simulink model "instrumentation_amplifier"  (R2020b)
settings: Solver=ode23t  StartTime=0.0  StopTime=4  RelTol=1e-3  EnableMultiTasking=on
libraries: fl_lib x10, ee_lib x7, nesl_utility x2
settings Model: Creator=lenovo  LastModifiedBy=bolic
settings DataIOCC: LimitDataPoints=on  SaveFormat=Array  SignalLoggingSaveFormat=ModelDataLogs  ReturnWorkspaceOutputs=off
settings OptimizationCC: ExpressionDepthLimit=2147483647  LifeSpan=inf
settings DebuggingCC: UnderspecifiedInitializationDetection=Classic  MergeDetectMultiDrivingBlocksExec=none  SolverPrmCheckMsg=warning  FcnCallInpInsideContextMsg=warning  StateNameClashWarn=warning  SFUnexpectedBacktrackingDiag=warning  SFNoUnconditionalDefaultTransitionDiag=warning  SFExecutionAtInitializationDiag=none  ArithmeticOperatorsInVariantConditions=warning
settings HardwareCC: ProdBitPerPointer=32  ProdBitPerSizeT=32  ProdBitPerPtrDiffT=32  ProdLargestAtomicFloat=None  ProdIntDivRoundTo=Undefined  ProdEndianess=Unspecified  ProdWordSize=32  ProdHWDeviceType=32-bit Generic
settings ModelReferenceCC: PropagateSignalLabelsOutOfModel=off
settings SFSimCC: SimUseLocalCustomCode=off  CustomCodeUndefinedFunction=UseInterfaceOnly
settings RTWCC: RTWUseLocalCustomCode=off
settings CodeAppCC: StateflowObjectComments=on
settings GRTTargetCC: TargetLangStandard=C89/C90 (ANSI)  CombineOutputUpdateFcns=off  GRTInterface=on
settings ConfigComp: CovMetricSettings=dw  CovSaveCumulativeToWorkspaceVar=on  CovSaveSingleToWorkspaceVar=on  CovExternalEMLEnable=off
settings SimscapeCC: SimscapeNormalizeSystem=off

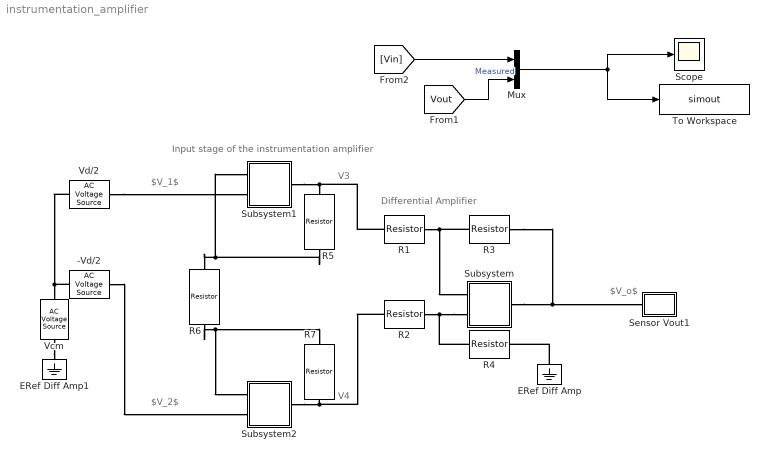
== system instrumentation_amplifier ==
  note: V4
  note: V3
  note: $V_o$
  note: Differential Amplifier
  note: Input stage of the instrumentation amplifier
  note: $V_1$
  note: $V_2$
  -Vd/2 : fl_lib/Electrical/Electrical Sources/AC Voltage Source  amp=0.02 V  shift=0 deg  frequency=1.2 Hz  omega=0 rad/s
  ERef Diff Amp : fl_lib/Electrical/Electrical Elements/Electrical Reference
      settings: SourceProductName=Foundation Library
  ERef Diff Amp1 : fl_lib/Electrical/Electrical Elements/Electrical Reference
      settings: SourceProductName=Foundation Library
  Mux : Mux  Inputs=2
  R1 : ee_lib/Passive/Resistor  R=1 kOhm  R_tol=1  enable_R_tol=0  tol_distribution=1  nSigma=4  enable_operating_limits=0  operating_limit_action=2  max_working_voltage=100 V  power_rating=1 W  enable_faults=0  fault_action=1  R_faulted=Inf Ohm  enable_temporal_fault=0  t_fault=1 s  enable_behavioral_fault=0  max_permissible_current=1 A  t_fail_on_current=1 s  noise_mode=0  sample_time=0.001 s  repeatability=1  auto_seed=2482559993  user_seed=0  Tdevice=25 degC  alpha=3.93e-3 1/K  Tmeas=25 degC  thermal_mass=100 J/K  power_derating_T1=70 degC  power_derating_T2=155 degC  operating_temperature_range_vec=[-50, 150] degC  temperature_specify=off  temperature_priority=High  temperature=298.15 K  temperature_nominal_specify=off  temperature_nominal_unit=K  temperature_nominal_value=1
  R2 : ee_lib/Passive/Resistor  R=1 kOhm  R_tol=1  enable_R_tol=0  tol_distribution=1  nSigma=4  enable_operating_limits=0  operating_limit_action=2  max_working_voltage=100 V  power_rating=1 W  enable_faults=0  fault_action=1  R_faulted=Inf Ohm  enable_temporal_fault=0  t_fault=1 s  enable_behavioral_fault=0  max_permissible_current=1 A  t_fail_on_current=1 s  noise_mode=0  sample_time=0.001 s  repeatability=1  auto_seed=854004048  user_seed=0  Tdevice=25 degC  alpha=3.93e-3 1/K  Tmeas=25 degC  thermal_mass=100 J/K  power_derating_T1=70 degC  power_derating_T2=155 degC  operating_temperature_range_vec=[-50, 150] degC  temperature_specify=off  temperature_priority=High  temperature=298.15 K  temperature_nominal_specify=off  temperature_nominal_unit=K  temperature_nominal_value=1
  R3 : ee_lib/Passive/Resistor  R=1 kOhm  R_tol=0.5  enable_R_tol=0  tol_distribution=1  nSigma=4  enable_operating_limits=0  operating_limit_action=2  max_working_voltage=100 V  power_rating=1 W  enable_faults=0  fault_action=1  R_faulted=Inf Ohm  enable_temporal_fault=0  t_fault=1 s  enable_behavioral_fault=0  max_permissible_current=1 A  t_fail_on_current=1 s  noise_mode=0  sample_time=0.001 s  repeatability=1  auto_seed=997392218  user_seed=0  Tdevice=25 degC  alpha=3.93e-3 1/K  Tmeas=25 degC  thermal_mass=100 J/K  power_derating_T1=70 degC  power_derating_T2=155 degC  operating_temperature_range_vec=[-50, 150] degC  temperature_specify=off  temperature_priority=High  temperature=298.15 K  temperature_nominal_specify=off  temperature_nominal_unit=K  temperature_nominal_value=1
  R4 : ee_lib/Passive/Resistor  R=1 kOhm  R_tol=1  enable_R_tol=0  tol_distribution=1  nSigma=4  enable_operating_limits=0  operating_limit_action=2  max_working_voltage=100 V  power_rating=1 W  enable_faults=0  fault_action=1  R_faulted=Inf Ohm  enable_temporal_fault=0  t_fault=1 s  enable_behavioral_fault=0  max_permissible_current=1 A  t_fail_on_current=1 s  noise_mode=0  sample_time=0.001 s  repeatability=1  auto_seed=1110524331  user_seed=0  Tdevice=25 degC  alpha=3.93e-3 1/K  Tmeas=25 degC  thermal_mass=100 J/K  power_derating_T1=70 degC  power_derating_T2=155 degC  operating_temperature_range_vec=[-50, 150] degC  temperature_specify=off  temperature_priority=High  temperature=298.15 K  temperature_nominal_specify=off  temperature_nominal_unit=K  temperature_nominal_value=1
  R5 : fl_lib/Electrical/Electrical Elements/Resistor  R=1 kOhm  i_specify=off  i_priority=None  i=0 A  i_nominal_specify=off  i_nominal_unit=A  i_nominal_value=1  v_specify=off  v_priority=None  v=0 V  v_nominal_specify=off  v_nominal_unit=V  v_nominal_value=1
  R6 : fl_lib/Electrical/Electrical Elements/Resistor  R=1 kOhm  i_specify=off  i_priority=None  i=0 A  i_nominal_specify=off  i_nominal_unit=A  i_nominal_value=1  v_specify=off  v_priority=None  v=0 V  v_nominal_specify=off  v_nominal_unit=V  v_nominal_value=1
  R7 : fl_lib/Electrical/Electrical Elements/Resistor  R=1 kOhm  i_specify=off  i_priority=None  i=0 A  i_nominal_specify=off  i_nominal_unit=A  i_nominal_value=1  v_specify=off  v_priority=None  v=0 V  v_nominal_specify=off  v_nominal_unit=V  v_nominal_value=1
  Scope : Scope
  Sensor Vout1 : Subsystem
      mask Display: disp('Vo')
  Subsystem : Subsystem
      mask Display: image('op_amp.png')
  Subsystem1 : Subsystem
      mask Display: image('op_amp.png')
  Subsystem2 : Subsystem
      mask Display: image('op_amp.png')
  To Workspace : ToWorkspace  VariableName=simout  SaveFormat=Timeseries  SampleTime=-1
  Vcm : fl_lib/Electrical/Electrical Sources/AC Voltage Source  amp=1 V  shift=0 deg  frequency=60 Hz  omega=0 rad/s
  Vd/2 : fl_lib/Electrical/Electrical Sources/AC Voltage Source  amp=0.02 V  shift=0 deg  frequency=1.2 Hz  omega=0 rad/s
  wires:
  Mux/1 -> To Workspace/1, Scope/1
  [Vin] -> Mux/1
  [Vout] -> Mux/2  "Measured"
  connections:
  Subsystem2/RConn1 -- R2/LConn1 -- R7/RConn1
  R6/RConn1 -- R7/LConn1 -- Subsystem2/LConn1
  Vd/2/RConn1 -- Subsystem1/LConn2
  Subsystem1/RConn1 -- R1/LConn1 -- R5/LConn1
  Subsystem/RConn1 -- R3/RConn1 -- Sensor Vout1/LConn1
  R1/RConn1 -- R3/LConn1 -- Subsystem/LConn1
  Subsystem/LConn2 -- R4/LConn1 -- R2/RConn1
  ERef Diff Amp/LConn1 -- R4/RConn1
  -Vd/2/RConn1 -- Subsystem2/LConn2
  Vcm/LConn1 -- Vd/2/LConn1 -- -Vd/2/LConn1
  Vcm/RConn1 -- ERef Diff Amp1/LConn1
  R6/LConn1 -- R5/RConn1 -- Subsystem1/LConn1

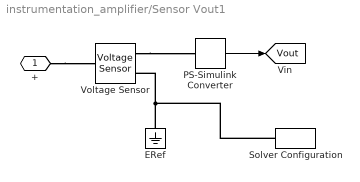
== system instrumentation_amplifier/Sensor Vout1 ==
  ERef : fl_lib/Electrical/Electrical Elements/Electrical Reference
      settings: SourceProductName=Foundation Library
  PS-Simulink Converter : nesl_utility/PS-Simulink Converter  PhysicalDomain=network_engine_domain  SubClassName=ps_output  LeftPortType=input  RightPortType=output  PseudoPeriodic=off  Frequencies=[]  Unit=1  AffineConversion=off
      settings: SourceProductName=Utilities
  Solver Configuration : nesl_utility/Solver Configuration  PhysicalDomain=network_engine_domain  SubClassName=solver  LeftPortType=input  RightPortType=generic  Tones=[]  Harmonics=[]  SimulateNoise=off  Profile=off  UseLocalSampling=off  EnableSwitchedLinearOptims=on  FrequencyDomain=off  UseCCode=off  RelTol=0.001  AbsTol=1e-06  MinStep=1e-09  ToWorkspace=off  RevertToSquareIcSolve=off  NumHomotopyIterations=100  PhasorMode=off  PhasorModeNumHarmonics=1  DoDC=off  ResidualTolerance=1e-9  UseLocalSolver=off  LocalSolverChoice=NE_BACKWARD_EULER_ADVANCER  LocalSolverSampleTime=.001  DoFixedCost=off  MaxNonlinIter=3  MaxModeIter=2  ComputeImpulses=off  ImpulseIterations=2  LinearAlgebra=auto  EquationFormulation=NE_TIME_EF  DelaysMemoryBudget=1024  AutomaticFiltering=on  FilteringTimeConstant=0.001  PartitionStorageMethod=AS_NEEDED  PartitionMemoryBudget=1024  PartitionMethod=FAST
  Voltage Sensor : fl_lib/Electrical/Electrical Sensors/Voltage Sensor
      settings: SourceProductName=Foundation Library
  + : PMIOPort  Side=Left
  tag scope: Vout=global
  wires:
  PS-Simulink Converter/1 -> [Vout]
  connections:
  ERef/LConn1 -- Solver Configuration/RConn1 -- Voltage Sensor/RConn2
  Voltage Sensor/RConn1 -- PS-Simulink Converter/LConn1
  +/RConn1 -- Voltage Sensor/LConn1

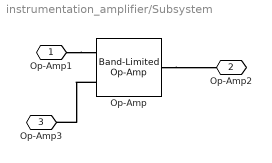
== system instrumentation_amplifier/Subsystem ==
  Op-Amp : ee_lib/Integrated Circuits/Band-Limited Op-Amp  A=1000  Rin=1e+06 Ohm  Rout=100 Ohm  Vmin=-15 V  Vmax=15 V  Vdotmax=1000 V/s  f=1e5 Hz  V0=0 V
      settings: SourceProductBaseCode=PS
  Op-Amp1 : PMIOPort  Side=Left
  Op-Amp2 : PMIOPort  Port=2  Side=Right
  Op-Amp3 : PMIOPort  Port=3  Side=Left
  connections:
  Op-Amp1/RConn1 -- Op-Amp/LConn2
  Op-Amp/LConn1 -- Op-Amp3/RConn1
  Op-Amp/RConn1 -- Op-Amp2/RConn1

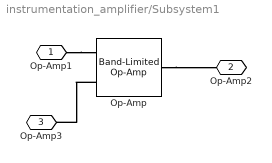
== system instrumentation_amplifier/Subsystem1 ==
  Op-Amp : ee_lib/Integrated Circuits/Band-Limited Op-Amp  A=1000  Rin=1e+09 Ohm  Rout=100 Ohm  Vmin=-15 V  Vmax=15 V  Vdotmax=1000 V/s  f=1e5 Hz  V0=0 V
      settings: SourceProductBaseCode=PS
  Op-Amp1 : PMIOPort  Side=Left
  Op-Amp2 : PMIOPort  Port=2  Side=Right
  Op-Amp3 : PMIOPort  Port=3  Side=Left
  connections:
  Op-Amp1/RConn1 -- Op-Amp/LConn2
  Op-Amp/LConn1 -- Op-Amp3/RConn1
  Op-Amp/RConn1 -- Op-Amp2/RConn1

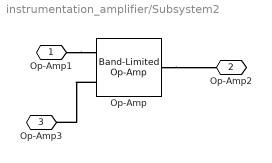
== system instrumentation_amplifier/Subsystem2 ==
  Op-Amp : ee_lib/Integrated Circuits/Band-Limited Op-Amp  A=1000  Rin=1e+09 Ohm  Rout=100 Ohm  Vmin=-15 V  Vmax=15 V  Vdotmax=1000 V/s  f=1e5 Hz  V0=0 V
      settings: SourceProductBaseCode=PS
  Op-Amp1 : PMIOPort  Side=Left
  Op-Amp2 : PMIOPort  Port=2  Side=Right
  Op-Amp3 : PMIOPort  Port=3  Side=Left
  connections:
  Op-Amp1/RConn1 -- Op-Amp/LConn2
  Op-Amp/LConn1 -- Op-Amp3/RConn1
  Op-Amp/RConn1 -- Op-Amp2/RConn1
